simulink model "AltitudeModeAutopilotMdlRef"  (R2018a)
settings: Solver=FixedStepDiscrete  StartTime=0.0  StopTime=25  FixedStep=1/40  RelTol=1e-3
libraries: aerolibconvert2 x2, simulink x2, LibraryAutopilot x1
settings Model: Creator=The MathWorks, Inc.  LastModifiedBy=The MathWorks, Inc.
settings DataIOCC: ExternalInput=rollIn  SaveFormat=StructureWithTime  SaveOutput=off  DSMLogging=off  SaveTime=off  OutputSaveName=Ail_Cmd  SignalLoggingName=Altitude_Mode_logsout
settings OptimizationCC: BlockReduction=off  DefaultParameterBehavior=Inlined  InlineInvariantSignals=on  EnhancedBackFolding=on  ExpressionDepthLimit=2147483647  EfficientFloat2IntCast=on  EfficientMapNaN2IntZero=off  LifeSpan=inf  MaxStackSize=inf
settings DebuggingCC: SignalInfNanChecking=error  SignalRangeChecking=error  ReadBeforeWriteMsg=EnableAllAsError  WriteAfterWriteMsg=EnableAllAsError  WriteAfterReadMsg=EnableAllAsError  AlgebraicLoopMsg=error  ArtificialAlgebraicLoopMsg=error  SaveWithDisabledLinksMsg=error  SaveWithParameterizedLinksMsg=error  CheckExecutionContextPreStartOutputMsg=on  CheckExecutionContextRuntimeOutputMsg=on  BlockPriorityViolationMsg=error  MaxConsecutiveZCsMsg=warning  SolverPrmCheckMsg=error  InheritedTsInSrcMsg=error  SingleTaskRateTransMsg=error  TasksWithSamePriorityMsg=error  SigSpecEnsureSampleTimeMsg=error  CheckMatrixSingularityMsg=error  IntegerOverflowMsg=error  ParameterUnderflowMsg=error  ParameterPrecisionLossMsg=error  ParameterTunabilityLossMsg=error  UnderSpecifiedDataTypeMsg=error  UnnecessaryDatatypeConvMsg=warning  VectorMatrixConversionMsg=error  SignalLabelMismatchMsg=error  UnconnectedInputMsg=error  UnconnectedOutputMsg=error  UnconnectedLineMsg=error  SFcnCompatibilityMsg=error  UniqueDataStoreMsg=error  BusObjectLabelMismatch=error  RootOutportRequireBusObject=error  AssertControl=DisableAll  AllowSymbolicDim=off  ModelReferenceIOMsg=error  ModelReferenceIOMismatchMessage=error  UnknownTsInhSupMsg=error  ModelReferenceDataLoggingMessage=error  ModelReferenceExtraNoncontSigs=none  StateNameClashWarn=warning  StrictBusMsg=ErrorOnBusTreatedAsVector  NonBusSignalsTreatedAsBus=error  SFUnexpectedBacktrackingDiag=warning  SFNoUnconditionalDefaultTransitionDiag=warning  SFExecutionAtInitializationDiag=none  IntegerSaturationMsg=error
settings HardwareCC: ProdBitPerPointer=32  ProdBitPerSizeT=32  ProdBitPerPtrDiffT=32  ProdLargestAtomicFloat=None  ProdEndianess=BigEndian  ProdWordSize=32  ProdHWDeviceType=32-bit Embedded Processor  TargetHWDeviceType=32-bit Generic
settings ModelReferenceCC: PropagateSignalLabelsOutOfModel=off
settings SFSimCC: MATLABDynamicMemAlloc=off
settings RTWCC: SystemTargetFile=ert.tlc  TemplateMakefile=ert_default_tmf  GenerateReport=on  RTWVerbose=off  IncludeHyperlinkInReport=on  LaunchReport=on  PortableWordSizes=on  GenerateTraceInfo=on  GenerateTraceReport=on  GenerateTraceReportSl=on  GenerateTraceReportSf=on  GenerateTraceReportEml=on
settings CodeAppCC: ForceParamTrailComments=on  IgnoreCustomStorageClasses=off  MaxIdLength=63  MangleLength=4  CustomSymbolStrType=$N$R$M  StateflowObjectComments=on  InternalIdentifier=Classic  ReqsInCode=on
settings ERTTargetCC: UtilityFuncGeneration=Shared location  MultiwordLength=2048  IncludeMdlTerminateFcn=off  GeneratePreprocessorConditionals=Disable all  SuppressErrorStatus=on  SupportAbsoluteTime=off  SupportNonFinite=off  SupportComplex=off  ParenthesesLevel=Maximum  InlinedParameterPlacement=NonHierarchical  MultiInstanceErrorCode=None  ERTCustomFileTemplate=example_file_process.tlc  PreserveExpressionOrder=on  PreserveIfCondition=on  ConvertIfToSwitch=off  SuppressUnreachableDefaultCases=off
settings ConfigComp: CovSaveName=covdata_pitchAP  CovMetricSettings=dcmtre  CovHTMLOptions=-aTS=1 -bRG=1 -bTC=1 -hTR=1 -nFC=0 -scm=1 -bcm=1  CovHtmlReporting=on  CovSaveCumulativeToWorkspaceVar=on  CovSaveSingleToWorkspaceVar=on  CovCumulativeVarName=covCumulativeData_pitchAP  CovCumulativeReport=on  CovReportOnPause=off  CovExternalEMLEnable=off

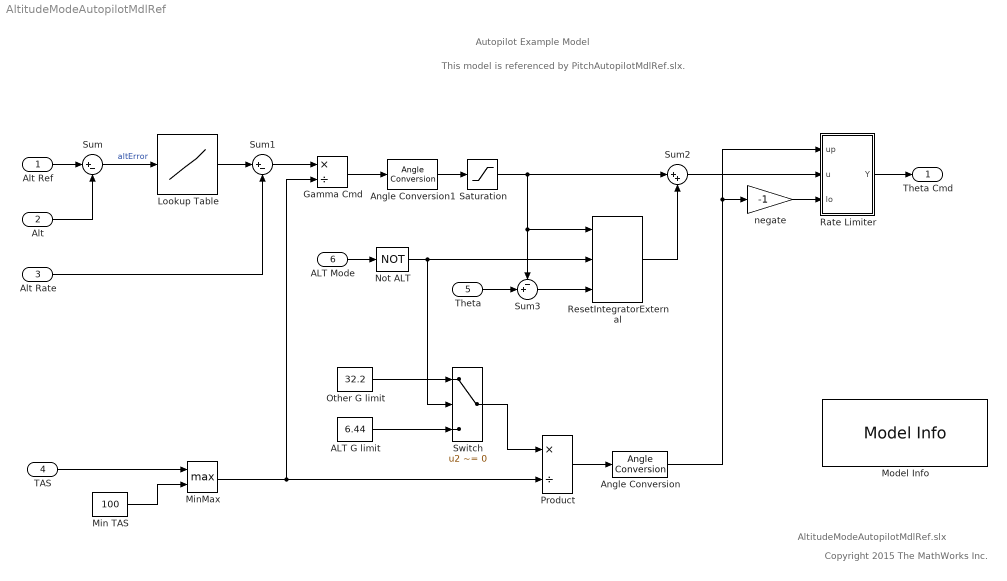
== system AltitudeModeAutopilotMdlRef ==
  note: Copyright 2015 The MathWorks Inc.
  note: AltitudeModeAutopilotMdlRef.slx
  note: This model is referenced by PitchAutopilotMdlRef.slx.
  note: Autopilot Example Model
  Alt Ref : Inport  OutDataTypeStr=double  PortDimensions=1  SampleTime=1/40  Interpolate=off
  Alt : Inport  Port=2  OutDataTypeStr=double  PortDimensions=1  SampleTime=1/40  Interpolate=off
  Alt Rate : Inport  Port=3  OutDataTypeStr=double  PortDimensions=1  SampleTime=1/40  Interpolate=off
  TAS : Inport  Port=4  OutDataTypeStr=double  PortDimensions=1  SampleTime=1/40  Interpolate=off
  Theta : Inport  Port=5  OutDataTypeStr=double  PortDimensions=1  SampleTime=1/40  Interpolate=off
  ALT Mode : Inport  Port=6  OutDataTypeStr=boolean  PortDimensions=1  SampleTime=1/40  Interpolate=off
  ALT G limit : Constant  Value=6.44  OutDataTypeStr=double
  Angle Conversion : aerolibconvert2/Angle Conversion  IU=rad  OU=deg
  Angle Conversion1 : aerolibconvert2/Angle Conversion  IU=rad  OU=deg
  Gamma Cmd : Product  Inputs=*/  RndMeth=Zero
  Lookup Table : Lookup_n-D  NumberOfTableDimensions=1  BreakpointsForDimension1=[-544 -206 -116 -52 0 52 116 206]  BreakpointsForDimension1FirstPoint=10  BreakpointsForDimension2FirstPoint=10  BreakpointsForDimension1Spacing=12  BreakpointsForDimension2Spacing=12  Table=[-42 -26 -19 -13 0 13 19 26]  ExtrapMethod=Clip  RemoveProtectionInput=on  UseLastTableValue=on  RndMeth=Zero  FractionDataTypeStr=double  InputSameDT=on
  Min TAS : Constant  Value=100  OutDataTypeStr=double
  MinMax : MinMax  Function=max  Inputs=2  InputSameDT=on
  Model Info : simulink/Model-Wide Utilities/Model Info  Frame=on  DisplayStringWithTags=|  HorizontalTextAlignment=Left  LeftAlignmentValue=0.02
      | Altitude Mode
      | Author: %<LastModifiedBy>
      | Version: %<ModelVersion>
      | Date: %<LastModificationDate>
  Not ALT : Logic  Operator=NOT  IconShape=distinctive  AllPortsSameDT=off  OutDataTypeStr=boolean
  Other G limit : Constant  Value=32.2  OutDataTypeStr=double
  Product : Product  Inputs=*/  RndMeth=Zero
  Rate Limiter : Subsystem  mask(Rate Limiter Dynamic){}
      mask Display: plot([0.15 0.95],[.5 .5],[.5 .5],[0.05 0.95],0.05+0.9*[.2 .8],0.05+0.9*[0 1]);
  ResetIntegratorExternal : LibraryAutopilot/ResetIntegratorExternal  K=0.2  Ts=1/40  UL=20
      settings: AttributesFormatString=K = %<K>\n-%<UL> to %<UL>  SourceProductName=Simulink Test  SourceProductBaseCode=SZ
  Saturation : Saturate  UpperLimit=20  LowerLimit=-20
  Sum : Sum  Inputs=|+-
  Sum1 : Sum  Inputs=|+-
  Sum2 : Sum  Inputs=|++
  Sum3 : Sum  Inputs=-+|
  Switch : Switch  Criteria=u2 ~= 0
  negate : Gain  Gain=-1
  Theta Cmd : Outport  OutDataTypeStr=double  PortDimensions=1  SampleTime=1/40
  wires:
  Other G limit/1 -> Switch/1
  ALT G limit/1 -> Switch/3
  Switch/1 -> Product/1
  Theta/1 -> Sum3/2
  Sum3/1 -> ResetIntegratorExternal/3
  ResetIntegratorExternal/1 -> Sum2/2
  ALT Mode/1 -> Not ALT/1
  Not ALT/1 -> ResetIntegratorExternal/2, Switch/2
  Angle Conversion1/1 -> Saturation/1
  Angle Conversion/1 -> negate/1, Rate Limiter/1(up)
  Product/1 -> Angle Conversion/1
  Sum2/1 -> Rate Limiter/2(u)
  Gamma Cmd/1 -> Angle Conversion1/1
  negate/1 -> Rate Limiter/3(lo)
  Sum1/1 -> Gamma Cmd/1
  Lookup Table/1 -> Sum1/1
  Rate Limiter/1(Y) -> Theta Cmd/1
  Sum/1 -> Lookup Table/1  "altError"
  Alt Ref/1 -> Sum/1
  Alt Rate/1 -> Sum1/2
  Alt/1 -> Sum/2
  MinMax/1 -> Gamma Cmd/2, Product/2
  TAS/1 -> MinMax/1
  Min TAS/1 -> MinMax/2
  Saturation/1 -> ResetIntegratorExternal/1, Sum3/1, Sum2/1

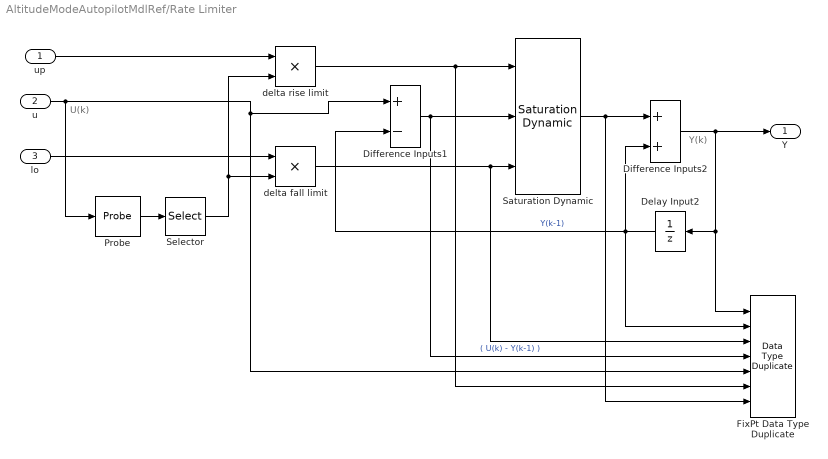
== system AltitudeModeAutopilotMdlRef/Rate Limiter ==
  note: Y(k)
  note: U(k)
  up : Inport
  u : Inport  Port=2
  lo : Inport  Port=3
  Delay Input2 : UnitDelay  Description=Store in Global RAM  DisableCoverage=on  SampleTime=-1
  Difference Inputs1 : Sum  Description=Add in CPU  DisableCoverage=on  Inputs=+-  OutDataTypeStr=Inherit: Inherit via back propagation
  Difference Inputs2 : Sum  Description=Add in CPU  OutDataTypeStr=Inherit: Inherit via back propagation
  FixPt Data Type Duplicate : DataTypeDuplicate  DisableCoverage=on  NumInputPorts=7
  Probe : Probe  ProbeWidth=off  ProbeComplexSignal=off
  Saturation Dynamic : simulink/Discontinuities/Saturation Dynamic  OutMin=[]  OutMax=[]  OutDataTypeStr=Inherit: Same as second input  OutDataType=fixdt(1, 16)  OutScaling=2^-10  DoSatur=off
  Selector : Selector  InputPortWidth=2  IndexOptions=Index vector (dialog)  Indices=[1]  OutputSizes=1
  delta fall limit : Product  DisableCoverage=on  Inputs=**  OutDataTypeStr=Inherit: Inherit via back propagation  SaturateOnIntegerOverflow=on
  delta rise limit : Product  DisableCoverage=on  Inputs=**  OutDataTypeStr=Inherit: Inherit via back propagation  SaturateOnIntegerOverflow=on
  Y : Outport  InitialOutput=0
  wires:
  Difference Inputs1/1 -> FixPt Data Type Duplicate/4, Saturation Dynamic/2  "( U(k) - Y(k-1) )"
  u/1 -> Probe/1, Difference Inputs1/1, FixPt Data Type Duplicate/5
  delta fall limit/1 -> FixPt Data Type Duplicate/3, Saturation Dynamic/3
  Saturation Dynamic/1 -> Difference Inputs2/1, FixPt Data Type Duplicate/7
  Delay Input2/1 -> Difference Inputs1/2, FixPt Data Type Duplicate/2, Difference Inputs2/2  "Y(k-1)"
  Difference Inputs2/1 -> Y/1, Delay Input2/1, FixPt Data Type Duplicate/1
  up/1 -> delta rise limit/1
  delta rise limit/1 -> FixPt Data Type Duplicate/6, Saturation Dynamic/1
  lo/1 -> delta fall limit/1
  Probe/1 -> Selector/1
  Selector/1 -> delta rise limit/2, delta fall limit/2
